simulink model "MPPT1"  (R2020a)
settings: Solver=VariableStepAuto  StartTime=0.0  StopTime=5  RelTol=1e-3
undefined symbols (not defined in the file): Ion, Lithium
libraries: powerlib x18, simulink x3, electricdrivelib x1, re_lib x1
settings Model: Creator=hp  LastModifiedBy=hp

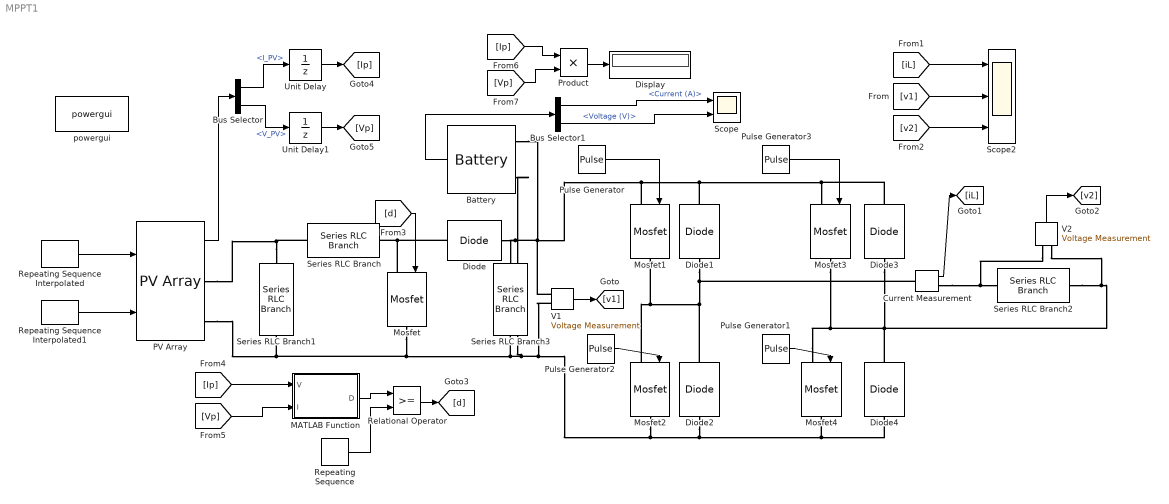
== system MPPT1 ==
  Battery : electricdrivelib/Extra Sources/Battery  BatType=Lithium-Ion  ShowTempParam=off  ThermalPreset=no  ShowAgeParam=off  NomV=900  NomQ=4000  SOC=66  Batt_Tr=.003  PresetModel=on  MaxQ=4000  MinV=675  FullV=1047.5884  Dis_rate=1739.1304  R=0.00225  Normal_OP=3617.3913  expZone="[972.3473      196.5217]"  current=[6.5 13 32.5]  Units=Time  Tci=20  NomT=20  T2=-30  MaxQ2=4.8  FullV2=7.1  Normal_OP2=5.655  expZone2="[6.58           1]"  Rca=0.6  ti=2000  Dp=0  Neq0=0  Tsim=1e6  Ta1=25  Qeol=5.4*0.9  Reol=0.013333*1.2  Char_age=[2.3478, 3]  Dis_age=[2.3478, 10]  N1=1500  N2=10500  N3=1000  N4=1400  Ta2=45  N5=950
  Bus Selector : BusSelector  OutputSignals=I_PV,V_PV
  Bus Selector1 : BusSelector  OutputSignals=Current (A),Voltage (V)
  Current Measurement : powerlib/Measurements/Current Measurement  PhasorSimulation=off  OutputType=Complex  PSBequivalent=0
  Diode{,1..4} (5 alike) : powerlib/Power Electronics/Diode  Ron=0.001  Lon=0  Vf=0.8  IC=0  UseSnubber=0  Rs=500  Cs=250e-9  Measurements=off
  Display : Display
  MATLAB Function : MATLAB Function  TreatAsAtomicUnit=on
  Mosfet{,1..4} (5 alike) : powerlib/Power Electronics/Mosfet  Ron=0.1  Lon=0  Rd=0.01  Vfd=0  IC=0  Rs=1e5  Cs=inf  Measurements=off
  PV Array : re_lib/Solar/PV Array  Npar=4  Nser=4  PlotType=array @ 1000 W/m2 & specified temperatures  S_vec="[ 1000  500  100 ]"  Temp_C_vec="[ 45 25  ]"  ModuleName=Centrosolar America BP7-315BW  PlotWhenSelected=off  Pm=315.0042  Ncell=72  Voc=45.45  Isc=8.97  Vm=37.59  Im=8.38  beta_Voc_pc=-0.349  alpha_Isc_pc=0.037001  beta_Voc=-0.15862  alpha_Isc=0.003319  IL=8.9803  I0=1.9823e-10  nI=1.0022  Rsh=237.0635  Rs=0.27147  RobustModel=off  RobustCellTemperature=25  BAL=on  Tc=1e-6  Tfilter=5e-5
  Product : Product
  Pulse Generator : DiscretePulseGenerator  PulseType=Time based  Period=1/(50)  PulseWidth=50  PhaseDelay=0/(360*50)
  Pulse Generator1 : DiscretePulseGenerator  PulseType=Time based  Period=1/(50)  PulseWidth=50  PhaseDelay=0/(360*50)
  Pulse Generator2 : DiscretePulseGenerator  PulseType=Time based  Period=1/(50)  PulseWidth=50  PhaseDelay=180/(360*50)
  Pulse Generator3 : DiscretePulseGenerator  PulseType=Time based  Period=1/(50)  PulseWidth=50  PhaseDelay=180/(360*50)
  Relational Operator : RelationalOperator  OutDataTypeStr=boolean  RndMeth=Simplest
  Repeating Sequence : simulink/Sources/Repeating Sequence  rep_seq_t=[0 1/(50e3)]  rep_seq_y=[0 1]
  Repeating Sequence Interpolated : simulink/Sources/Repeating Sequence Interpolated  OutValues=[100 300 400 600 1000 1000 800 200]  TimeValues=[0 .1 .2 .3 .4 4 4.8 5]  LookUpMeth=Interpolation-Use End Values  tsamp=.0001  OutMin=[]  OutMax=[]  OutDataTypeStr=double  OutputDataTypeScalingMode=double  OutDataType=fixdt(0,8)  OutScaling=2^-10
  Repeating Sequence Interpolated1 : simulink/Sources/Repeating Sequence Interpolated  OutValues=[15 18 22 23 25 25 21 12]  TimeValues=[0 .1 .2 .3 .4 4 4.8 5]  LookUpMeth=Interpolation-Use End Values  tsamp=0.0001  OutMin=[]  OutMax=[]  OutDataTypeStr=double  OutputDataTypeScalingMode=double  OutDataType=fixdt(0,8)  OutScaling=2^-10
  Scope : Scope  NumInputPorts=2
  Scope2 : Scope  NumInputPorts=3
  Series RLC Branch : powerlib/Elements/Series RLC Branch  LConnTagsString=__new0  RConnTagsString=__new0  BranchType=L  Resistance=1  Inductance=0.0021  SetiL0=off  InitialCurrent=0  Capacitance=1e-6  Setx0=off  InitialVoltage=0  Measurements=None
  Series RLC Branch1 : powerlib/Elements/Series RLC Branch  LConnTagsString=__new0  RConnTagsString=__new0  BranchType=C  Resistance=1  Inductance=1e-3  SetiL0=off  InitialCurrent=0  Capacitance=1.2817e-04  Setx0=off  InitialVoltage=0  Measurements=None
  Series RLC Branch2 : powerlib/Elements/Series RLC Branch  LConnTagsString=__new0  RConnTagsString=__new0  BranchType=R  Resistance=181.6700  Inductance=1e-3  SetiL0=off  InitialCurrent=0  Capacitance=1e-6  Setx0=off  InitialVoltage=0  Measurements=None
  Series RLC Branch3 : powerlib/Elements/Series RLC Branch  LConnTagsString=__new0  RConnTagsString=__new0  BranchType=C  Resistance=1  Inductance=1e-3  SetiL0=off  InitialCurrent=0  Capacitance=1.8558e-05  Setx0=off  InitialVoltage=0  Measurements=None
  Unit Delay : UnitDelay  SampleTime=1e-4  HasFrameUpgradeWarning=on
  Unit Delay1 : UnitDelay  SampleTime=1e-4  HasFrameUpgradeWarning=on
  V1 : powerlib/Measurements/Voltage Measurement  PhasorSimulation=off  OutputType=Complex  PSBequivalent=0
  V2 : powerlib/Measurements/Voltage Measurement  PhasorSimulation=off  OutputType=Complex  PSBequivalent=0
  powergui : powerlib/powergui  Priority=1  SimulationMode=Discrete  SampleTime=50e-8  frequency=60  Iterations=50  frequencyindice=0  Pbase=100e6  ErrMax=1e-4  UnitsV=kV  UnitsW=MW  buscounter=0  FunctionMessages=off  echomessages=off  EnableUseOfTLC=off  CurrentSourceSwitches=off  DisableSnubberDevices=off  DisableRonSwitches=off  DisableVfSwitches=off  DisplayEquations=off  AutomaticDiscreteSolvers=off  SolverType=Tustin/Backward Euler (TBE)  Interpol=off  ExternalGateDelay=off  methode=off  Ts=100  x0status=blocks  SPID=on  SwTol=0  HookPort=off  NonlinearTolerance=1e-4  nMaxIteration=100  ContinueOnMaxIteration=off  RestoreLinks=warning  ResistiveCurrentMeasurement=off  Frange=[0:2:500]  Ylog=off  Xlog=on  ShowGrid=off  save=off  variable=ZData  structure=0  ZoomFFT=off  StartTime=0.0  cycles=1  DisplayStyle=1  fundamental=60  FreqAxis=off  MaxFrequency=1000  frequencyindicesteady=1  RmsSteady=1  display=off
  wires:
  [Ip] -> Product/1
  Bus Selector/2 -> Unit Delay1/1  "<V_PV>"
  Bus Selector/1 -> Unit Delay/1  "<I_PV>"
  Current Measurement/1 -> [iL]
  Unit Delay/1 -> [Ip]
  PV Array/1 -> Bus Selector/1
  [iL] -> Scope2/1
  Relational Operator/1 -> [d]
  Pulse Generator/1 -> Mosfet1/1
  Pulse Generator1/1 -> Mosfet4/1
  Product/1 -> Display/1
  Unit Delay1/1 -> [Vp]
  [v1] -> Scope2/2
  [v2] -> Scope2/3
  Pulse Generator3/1 -> Mosfet3/1
  Pulse Generator2/1 -> Mosfet2/1
  V1/1 -> [v1]
  [d] -> Mosfet/1
  MATLAB Function/1(D) -> Relational Operator/1
  V2/1 -> [v2]
  [Vp] -> MATLAB Function/2(I)
  [Vp] -> Product/2
  [Ip] -> MATLAB Function/1(V)
  Repeating Sequence Interpolated/1 -> PV Array/1
  Repeating Sequence/1 -> Relational Operator/2
  Repeating Sequence Interpolated1/1 -> PV Array/2
  Battery/1 -> Bus Selector1/1
  Bus Selector1/1 -> Scope/1  "<Current (A)>"
  Bus Selector1/2 -> Scope/2  "<Voltage (V)>"
  connections:
  Diode1/LConn1 -- Diode2/RConn1 -- Mosfet2/LConn1 -- Mosfet1/RConn1 -- Current Measurement/LConn1
  Mosfet1/LConn1 -- Mosfet3/LConn1 -- Diode3/RConn1 -- Diode1/RConn1 -- Diode/RConn1 -- Series RLC Branch3/LConn1 -- Battery/LConn1 -- V1/LConn1
  Diode/LConn1 -- Series RLC Branch/RConn1 -- Mosfet/LConn1
  Series RLC Branch3/RConn1 -- Battery/LConn2 -- V1/LConn2 -- Diode2/LConn1 -- Diode4/LConn1 -- Mosfet4/RConn1 -- Mosfet2/RConn1 -- Series RLC Branch1/RConn1 -- PV Array/RConn2 -- Mosfet/RConn1
  Series RLC Branch1/LConn1 -- Series RLC Branch/LConn1 -- PV Array/RConn1
  Mosfet4/LConn1 -- Diode3/LConn1 -- Series RLC Branch2/RConn1 -- V2/LConn2 -- Diode4/RConn1 -- Mosfet3/RConn1
  V2/LConn1 -- Series RLC Branch2/LConn1 -- Current Measurement/RConn1

== matlab function MPPT1/MATLAB Function ==
  data: V input; D output; I input
function D = Duty_cycle(V,I)
Dmax=.8429;
Dmim=.3675;
Dinit=.8429;
DelD=.0001;
persistent Vold Pold Dold;
datatype='double';

if isempty(Vold)
    Vold = 0;
    Pold = 0;
    Dold = Dinit;
end
P=V*I;
dV=V-Vold;
dP=P-Pold;
if dP~=0; % dP is not equel to zero
 if dP<0;
     if dV<0;
       D=Dold-DelD;
     else
       D=Dold+DelD;
     end
 else
     if dV<0;
       D=Dold+DelD;
     else
       D=Dold-DelD;
     end 
 end
else 
    D=Dold;
end
if D>=Dmax || D<Dmim
    D=Dold;
end
Dold=D;
Vold=V;
Pold=P;
